simulink library "CTRL_TRGT_DEC"  (R2023b)
settings: Solver=VariableStepAuto  StartTime=0.0  StopTime=10.0  RelTol=1e-3
settings Model: Creator=blatak  LastModifiedBy=blatak

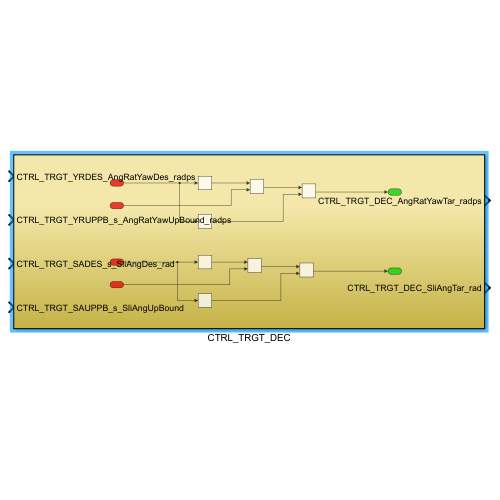
[thumbnail: Simulink's stored preview of the top-level diagram]
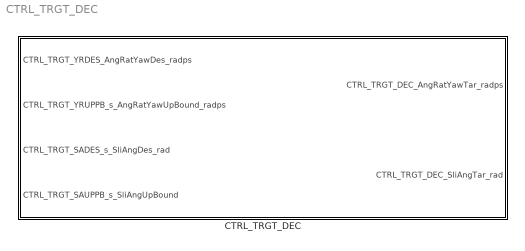
== system CTRL_TRGT_DEC ==
  CTRL_TRGT_DEC : Subsystem

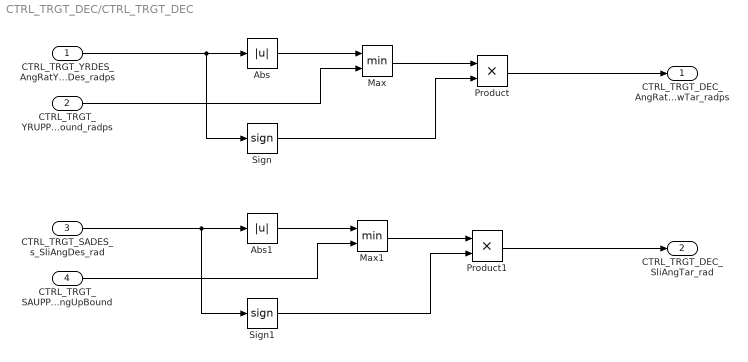
== system CTRL_TRGT_DEC/CTRL_TRGT_DEC ==
  CTRL_TRGT_YRDES_AngRatYawDes_radps : Inport
  CTRL_TRGT_YRUPPB_s_AngRatYawUpBound_radps : Inport  Port=2
  CTRL_TRGT_SADES_s_SliAngDes_rad : Inport  Port=3
  CTRL_TRGT_SAUPPB_s_SliAngUpBound : Inport  Port=4
  Abs : Abs  SaturateOnIntegerOverflow=off
  Abs1 : Abs  SaturateOnIntegerOverflow=off
  Max : MinMax  Inputs=2
  Max1 : MinMax  Inputs=2
  Product : Product
  Product1 : Product
  Sign : Signum
  Sign1 : Signum
  CTRL_TRGT_DEC_AngRatYawTar_radps : Outport
  CTRL_TRGT_DEC_SliAngTar_rad : Outport  Port=2
  wires:
  Product/1 -> CTRL_TRGT_DEC_AngRatYawTar_radps/1
  Max1/1 -> Product1/1
  Max/1 -> Product/1
  Sign/1 -> Product/2
  CTRL_TRGT_SADES_s_SliAngDes_rad/1 -> Abs1/1, Sign1/1
  CTRL_TRGT_SAUPPB_s_SliAngUpBound/1 -> Max1/2
  Sign1/1 -> Product1/2
  CTRL_TRGT_YRUPPB_s_AngRatYawUpBound_radps/1 -> Max/2
  CTRL_TRGT_YRDES_AngRatYawDes_radps/1 -> Abs/1, Sign/1
  Abs1/1 -> Max1/1
  Abs/1 -> Max/1
  Product1/1 -> CTRL_TRGT_DEC_SliAngTar_rad/1
